simulink library "pmm"  (R2021b)
settings: Solver=VariableStepAuto  StartTime=0.0  StopTime=10.0  RelTol=1e-3
undefined symbols (not defined in the file): APMM_CoolgFanActCurr_X_pct, APMM_EWP1Curr_X_c, APMM_EWP3Curr_X_c, APMM_LVBattChktime_X_enum, APMM_LVBattChrgtime_X_enum, APMM_LVChrgLv_X_mV, ENUM_ANTITHEFT_ALARM, ENUM_ANTITHEFT_ARM, ENUM_ANTITHEFT_DISARM, ENUM_ANTITHEFT_WAIT, ENUM_APSSYSTEMSTA_REMOTEACTIVE, ENUM_CHRGPLUGSTA_NONE, ENUM_CRASHSTATE_FRONTFIRSTLV, ENUM_CRASHSTATE_LEFTSIDE, ENUM_CRASHSTATE_RIGHTSIDE, ENUM_DRIVETRAIN_AWD, ENUM_DRIVETRAIN_FWD, ENUM_DRIVETRAIN_RWD, ENUM_DRSEATSTA_EMPTY, ENUM_DRSEATSTA_INVALID, ENUM_DRSEATSTA_OCCUPIED, ENUM_EPBSTA_APPLIED, ENUM_GEARACTUALPOSN_D, ENUM_GEARACTUALPOSN_N, ENUM_GEARACTUALPOSN_P, ENUM_GEARACTUALPOSN_R, ENUM_HVBATTREADYPRE_READY, ENUM_OTACHKSTA_NOREQUEST, ENUM_OTACHKSTA_NOTIMEOUT, ENUM_OTACHKSTA_TIMEOUT, ENUM_PDKEYRAWLULOCK_INLOCK, ENUM_PDKEYRAWLULOCK_INUNLOCK, ENUM_PDKEYRAWPS_INPS, ENUM_PDKEYSTA_LOCK, ENUM_PDKEYSTA_PS, ENUM_PDKEYSTA_UNAVALIABLE, ENUM_PDKEYSTA_UNLOCK, ENUM_POWERSTA_OFF, ENUM_POWERSTA_OFFC, ENUM_POWERSTA_STANDBY, ENUM_PWRREQOTA_NOREQUEST, ENUM_PWRREQOTA_REQPOWEROFF, ENUM_PWRREQOTA_REQPOWERSTDBY, ENUM_PWRSTASW_READY, ENUM_V2LSTA_NOPLUG, ENUM_VEHICLETYPE_D31L24, ENUM_VEHMALFUNLEVEL_LEVEL3, ENUM_VEHMALFUNLEVEL_LEVEL4, FALSE, KPMM_AllDoorClosedHoldTime_s, KPMM_APSAllowThd_pct, KPMM_BattDownFailtime_s, KPMM_BattUpFailtime_s, KPMM_BattUpResetRty_cnt, KPMM_BattUpResetSW_flg, KPMM_BattUpResetTO_s, KPMM_BattUpRstDlyTO_s, KPMM_BrakeSWHoldTime_s, KPMM_CANValidChkFailtime_s, KPMM_ChrgPlugHoldTime_s ... (+87)
libraries: simulink x29, hcu_lib x24
(part 4 of 7)

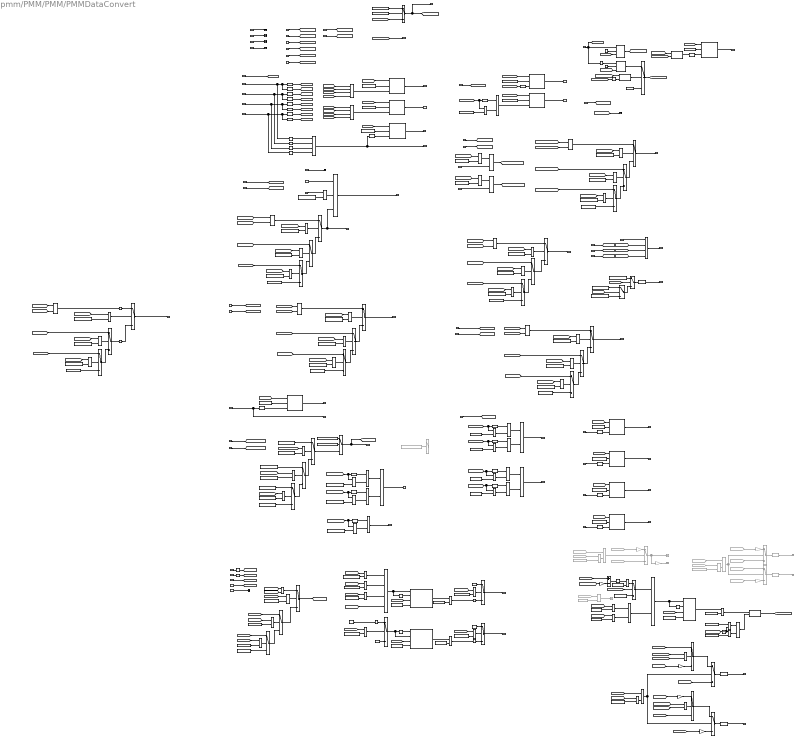
== system pmm/PMM/PMM/PMMDataConvert ==
  note: Detect HV power state
  note: Detect PW Continue Use
  note: Detect SchedChgwake
  note: Detect IVI Power OFF
  note: Monitor for DCDC fault level
  note: Safety Check
  note: 0 = HVIL close; 1 = HVIL open
  note: Seat Switch Rising Edge
  note: Detect Gun Plug Rising/Faling Edge
  note: KEY STATE
  note: Brake signal convert to rising edge
  note: Door judgement
  note: Precharge Check
  note: MCU Enable
  note: MCU Discharge
  note: MCU Ready
  note: Antitheft State
  note: OPDS Signal tramsmit function
  note: BMSWarn judgement
  note: MCU DC Bus Max Voltage judgement
  note: VPMM_SafetyChkHLv_flg
      | 0 Fail
      | 1 OK
  note: VPMM_TMSpdThdSta_flg
      | 0 = Not allow MCU disable
      | 1 = Allow MCU disable
  note: 0 = No fail;
      | 1 = fail
  note: VPMM_SafetyChkMLv_flg
      | 0 Fail
      | 1 OK
  note: Aux Battery Handle
  note: Comment out to reduce CPU resource.
      | Use below if judgement to avoid float multiply.
  note: MCU Disable
  task_time_s : Inport
  VBCM_AntitheftSta_enum : Inport  Port=2
  VINP_DrDoorSW_flg : Inport  Port=3
  VINP_PsDoorSW_flg : Inport  Port=4
  VINP_RRDoorSW_flg : Inport  Port=5
  VINP_RLDoorSW_flg : Inport  Port=6
  VINP_BrakeSWGPIO_flg : Inport  Port=7
  VINP_FrMCUDCBusVolt_V : Inport  Port=8
  VINP_FrMCUDischrgSta_flg : Inport  Port=9
  VINP_FrMCUEnaSta_flg : Inport  Port=10
  VINP_FrMCUErr_enum : Inport  Port=11
  VINP_FrMCUReady4Pre_flg : Inport  Port=12
  VINP_FrMCUReady_flg : Inport  Port=13
  VINP_FrMCUTemp_C : Inport  Port=14
  VINP_RrMCUDCBusVolt_V : Inport  Port=15
  VINP_RrMCUDischrgSta_flg : Inport  Port=16
  VINP_RrMCUEnaSta_flg : Inport  Port=17
  VINP_RrMCUErr_enum : Inport  Port=18
  VINP_RrMCUReady4Pre_flg : Inport  Port=19
  VINP_RrMCUReady_flg : Inport  Port=20
  VINP_RrMCUTemp_C : Inport  Port=21
  VINP_DCDCReady4Pre_flg : Inport  Port=22
  VINP_OBCReady4Pre_flg : Inport  Port=23
  VINP_HVBattReady4Pre_enum : Inport  Port=24
  VINP_PDKeyAreaPS_enum : Inport  Port=25
  VINP_PDKeyAreaLockUnlock_enum : Inport  Port=26
  VINP_ChrgPlugSta_enum : Inport  Port=27
  VINP_SeatSW_flg : Inport  Port=28
  VINP_HVILSta_flg : Inport  Port=29
  VINP_CrashOutputSts_enum : Inport  Port=30
  VPMM_PowerSta_enum : Inport  Port=31
  VINP_RrTMSpd_rpm : Inport  Port=32
  VINP_FrTMSpd_rpm : Inport  Port=33
  VINP_BMSWarn5_flg : Inport  Port=34
  VINP_BMSWarn6_flg : Inport  Port=35
  VINP_BMSWarn7_flg : Inport  Port=36
  VINP_BMSWarn8_flg : Inport  Port=37
  VINP_DrivetrainSelect_enum : Inport  Port=38
  VINP_DCDCFaultSta_enum : Inport  Port=39
  VINP_IVIPwroffreq_flg : Inport  Port=40
  VINP_SchedChgwake_flg : Inport  Port=41
  VINP_PWCONTINUEUSE_flg : Inport  Port=42
  VPMM_HVPwrSta_flg : Inport  Port=43
  VINP_LVBattDet12V_V : Inport  Port=44
  VINP_AuxBattVolmV_mV : Inport  Port=45
  VINP_NewNMSpec_flg : Inport  Port=46
  VINP_VehicleType_enum : Inport  Port=47
  VINP_CANMsgValidBMS5_flg : Inport  Port=48
  VTQD_CrashDetd_flg : Inport  Port=49
  VDDM_DrStSWCFS_flg : Inport  Port=50
  AND{,3..6,8} (6 alike) : Logic  AllPortsSameDT=off  OutDataTypeStr=boolean
  AND1 : Logic  Inputs=3  AllPortsSameDT=off  OutDataTypeStr=boolean
  AND2 : Logic  Operator=OR  AllPortsSameDT=off  OutDataTypeStr=boolean
  AND7 : Logic  Operator=OR  Inputs=4  AllPortsSameDT=off  OutDataTypeStr=boolean
  Abs : Abs
  Abs1 : Abs
  Abs2 : Abs
  Add : Sum  Inputs=+-
  Constant : Constant  Value=KPMM_DoorSWHoldTime_s
  Constant1 : Constant  Value=KPMM_DoorSWHoldTime_s
  Constant10 : Constant  Commented=on  Value=ENUM_VEHICLETYPE_D31L24
  Constant{4,11,19,22,30,38,84} (7 alike) : Constant  Value=ENUM_DRIVETRAIN_AWD
  Constant12 : Constant  Commented=on  Value=ENUM_VEHICLETYPE_D31L24
  Constant{6,13,21,32,39,46,85} (7 alike) : Constant  Value=ENUM_DRIVETRAIN_FWD
  Constant14 : Constant  Value=ENUM_HVBATTREADYPRE_READY
  Constant{8,15,23,34,40,51,86} (7 alike) : Constant  Value=ENUM_DRIVETRAIN_RWD
  Constant{7,9,16..17,28,55,82,87,93} (9 alike) : Constant  Value=FALSE
  Constant18 : Constant  Value=KPMM_ChrgPlugHoldTime_s
  Constant2 : Constant  Value=ZERO_FLOAT
  Constant20 : Constant  Value=KPMM_ChrgPlugHoldTime_s
  Constant24 : Constant  Value=KPMM_RrMCUDischrgVolt_V
  Constant25 : Constant  Value=KPMM_FrMCUDischrgVolt_V
  Constant26 : Constant  Value=KPMM_DrivetrainSelect_enum_ovrdflg
  Constant27 : Constant  Commented=on  Value=FALSE
  Constant29 : Constant  Value=ENUM_VEHICLETYPE_D31L24
  Constant3 : Constant  Value=KPMM_SeatSWHoldTime_s
  Constant31 : Constant  Value=ENUM_CHRGPLUGSTA_NONE
  Constant33 : Constant  Value=KPMM_LVADCUpThd_mV  OutDataTypeStr=uint16
  Constant35 : Constant  Value=ENUM_POWERSTA_STANDBY  OutDataTypeStr=uint8
  Constant36 : Constant  Value=KPMM_LVADCDiffThd_mV  OutDataTypeStr=uint16
  Constant37 : Constant  Value=KPMM_AllDoorClosedHoldTime_s
  Constant41 : Constant  Value=KPMM_BrakeSWHoldTime_s
  Constant42 : Constant  Value=KPMM_PDKeySta_enum_ovrdval
  Constant43 : Constant  Value=ENUM_PDKEYRAWPS_INPS
  Constant44 : Constant  Value=KPMM_PDKeySta_enum_ovrdflg
  Constant45 : Constant  Value=ENUM_PDKEYRAWLULOCK_INUNLOCK
  Constant47 : Constant  Value=ENUM_PDKEYRAWLULOCK_INLOCK
  Constant48 : Constant  Value=ENUM_PDKEYSTA_UNAVALIABLE
  Constant49 : Constant  Value=ENUM_PDKEYSTA_LOCK
  Constant5 : Constant  Value=ENUM_CRASHSTATE_FRONTFIRSTLV
  Constant50 : Constant  Value=ENUM_PDKEYSTA_UNLOCK
  Constant52 : Constant  Value=KPMM_DrivetrainSelect_enum_ovrdval
  Constant53 : Constant  Value=ENUM_ANTITHEFT_DISARM
  Constant54 : Constant  Value=ENUM_ANTITHEFT_WAIT
  Constant56 : Constant  Value=ENUM_PDKEYSTA_PS
  Constant57 : Constant  Value=KPMM_LVADCLoThd_mV  OutDataTypeStr=uint16
  Constant58 : Constant  Value=ENUM_PDKEYSTA_UNLOCK
  Constant59 : Constant  Value=ENUM_PDKEYSTA_PS
  Constant60 : Constant  Value=ENUM_ANTITHEFT_ARM
  Constant61 : Constant  Value=ENUM_ANTITHEFT_ALARM
  Constant62 : Constant  Value=ENUM_PDKEYSTA_LOCK
  Constant63 : Constant  Value=KPMM_IVIPwroffHoldTime_s
  Constant64 : Constant  Value=KPMM_SchedChgHoldTime_s
  Constant65 : Constant  Value=KPMM_PWCONTINUEHoldTime_s
  Constant66 : Constant  Value=KPMM_HVPwrStaHoldTime_s
  Constant67 : Constant  Value=ENUM_CRASHSTATE_RIGHTSIDE
  Constant68 : Constant  Value=ENUM_CRASHSTATE_LEFTSIDE
  Constant69 : Constant  Value=KPMM_TMSpdMCUDisThrsh_rpm
  Constant70 : Constant  Value=TRUE
  Constant71 : Constant  Value=KPMM_SaftyChkHLvTO_s
  Constant72 : Constant  Value=ENUM_POWERSTA_OFF
  Constant73 : Constant  Value=TRUE
  Constant74 : Constant  Value=KPMM_SaftyChkMLvTO_s
  Constant75 : Constant  Value=KPMM_SaftyChkMLvTO_s
  Constant76 : Constant  Value=TRUE
  Constant77 : Constant  Value=ENUM_POWERSTA_OFF
  Constant78 : Constant  Value=KPMM_LVADCErrTO_s  OutDataTypeStr=single
  Constant79 : Constant  Value=KPMM_SaftyChkHLvTO_s
  Constant80 : Constant  Value=ENUM_POWERSTA_OFF  OutDataTypeStr=uint8
  Constant81 : Constant  Commented=on  Value=0xFFFF  OutDataTypeStr=uint16
  Constant83 : Constant  Value=KPMM_LVADCErrTO_s  OutDataTypeStr=single
  Constant88 : Constant  Value=ENUM_DRSEATSTA_OCCUPIED
  Constant89 : Constant  Value=ENUM_DRSEATSTA_EMPTY
  Constant90 : Constant  Value=ENUM_DRSEATSTA_INVALID
  Constant91 : Constant  Value=200
  Constant92 : Constant  Value=2000
  Data Type Conversion : DataTypeConversion  OutDataTypeStr=uint8
  Data Type Conversion1 : DataTypeConversion  Commented=on
  Data Type Conversion2 : DataTypeConversion
  Data Type Conversion3 : DataTypeConversion  Commented=on
  Data Type Conversion4 : DataTypeConversion
  Delay : Delay  DelayLength=1
  DelayEnable : hcu_lib/Basic_Blocks/DelayEnable
  DelayEnable1 : hcu_lib/Basic_Blocks/DelayEnable
  Detect Change{,1..6} (7 alike) : simulink/Logic and Bit Operations/Detect Change  vinit=0  OutDataTypeStr=boolean
  Detect Decrease{,1..4} (5 alike) : simulink/Logic and Bit Operations/Detect Decrease  vinit=0.0  OutDataTypeStr=boolean
  Detect Increase{,1..11} (12 alike) : simulink/Logic and Bit Operations/Detect Increase  vinit=0.0  OutDataTypeStr=boolean
  Equal{,1..9,12,14..18,20..22,24..25,27..38,41,44,50..52} (38 alike) : RelationalOperator  Operator===  OutDataTypeStr=boolean  RndMeth=Simplest
  Equal10 : RelationalOperator  Operator=<=  OutDataTypeStr=boolean  RndMeth=Simplest
  Equal11 : RelationalOperator  Operator=<=  OutDataTypeStr=boolean  RndMeth=Simplest
  Equal13 : RelationalOperator  Commented=on  Operator=~=  OutDataTypeStr=boolean  RndMeth=Simplest
  Equal19 : RelationalOperator  Operator=~=  OutDataTypeStr=boolean  RndMeth=Simplest
  Equal23 : RelationalOperator  Commented=on  Operator===  OutDataTypeStr=boolean  RndMeth=Simplest
  Equal26 : RelationalOperator  Commented=on  Operator=~=  OutDataTypeStr=boolean  RndMeth=Simplest
  Equal{39..40,42,47..48} (5 alike) : RelationalOperator  OutDataTypeStr=boolean  RndMeth=Simplest
  Equal43 : RelationalOperator  Operator=<  OutDataTypeStr=boolean  RndMeth=Simplest
  Equal45 : RelationalOperator  Operator=~=  OutDataTypeStr=boolean  RndMeth=Simplest
  Equal46 : RelationalOperator  Operator=~=  OutDataTypeStr=boolean  RndMeth=Simplest
  Equal49 : RelationalOperator  Operator=<=  OutDataTypeStr=boolean  RndMeth=Simplest
  From100 : From  Commented=on  GotoTag=VINP_LVBattDet12V_V
  From{95,101..102,117} (4 alike) : From  Commented=on  GotoTag=VINP_AuxBattVolmV_mV
  From93 : From  Commented=on  GotoTag=VINP_VehicleType_enum
  From94 : From  Commented=on  GotoTag=VINP_NewNMSpec_flg
  From96 : From  Commented=on  GotoTag=VINP_LVBattDet12V_V
  From97 : From  Commented=on  GotoTag=VINP_VehicleType_enum
  From98 : From  Commented=on  GotoTag=VINP_NewNMSpec_flg
  From99 : From  Commented=on  GotoTag=VINP_LVBattDet12V_V
  Gain : Gain  Commented=on  Gain=1000
  Gain1 : Gain  Commented=on  Gain=0.001
  Gain2 : Gain  Commented=on  Gain=0.001
  Gain3 : Gain  Commented=on  Gain=1000
  Gain4 : Gain  Gain=1000
  Gain5 : Gain  Gain=0.001
  Gain6 : Gain  Gain=1000
  Gain7 : Gain  Gain=1000
  Hold{,1..10} (11 alike) : hcu_lib/Basic_Blocks/Hold  SystemSampleTime=-1  VariantActivationTime=update diagram  Latency=0  AutoFrameSizeCalculation=off
      settings: SourceProductName=HCU Relative Block Library
  LiuzgSwitch{1..18,22..32} (29 alike) : Switch  Criteria=u2 ~= 0
      settings: AttributesFormatString=<%<Criteria>>
  LiuzgSwitch19 : Switch  Commented=on  Criteria=u2 ~= 0
      settings: AttributesFormatString=<%<Criteria>>
  LiuzgSwitch20 : Switch  Commented=on  Criteria=u2 ~= 0
      settings: AttributesFormatString=<%<Criteria>>
  LiuzgSwitch21 : Switch  Commented=on  Criteria=u2 ~= 0
      settings: AttributesFormatString=<%<Criteria>>
  Logical Operator : Logic  Operator=NOT  AllPortsSameDT=off  OutDataTypeStr=boolean
  Logical Operator{1..3,5..6,8..9,11,15..17,20} (12 alike) : Logic  AllPortsSameDT=off  OutDataTypeStr=boolean
  Logical Operator{4,7,10,18..19} (5 alike) : Logic  Operator=OR  AllPortsSameDT=off  OutDataTypeStr=boolean
  Logical Operator12 : Logic  Commented=on  AllPortsSameDT=off  OutDataTypeStr=boolean
  Logical Operator13 : Logic  Operator=OR  Inputs=4  AllPortsSameDT=off  OutDataTypeStr=boolean
  Logical Operator14 : Logic  Commented=on  AllPortsSameDT=off  OutDataTypeStr=boolean
  Logical Operator21 : Logic  Operator=NOT  AllPortsSameDT=off  OutDataTypeStr=boolean
  Logical Operator22 : Logic  Operator=NOT  AllPortsSameDT=off  OutDataTypeStr=boolean
  Max : MinMax  Function=max  Inputs=2
  Max1 : MinMax  Function=max  Inputs=2
  NOT{1..9,11} (10 alike) : Logic  Operator=NOT  AllPortsSameDT=off  OutDataTypeStr=boolean
  OR : Logic  Operator=OR  Inputs=4  AllPortsSameDT=off  OutDataTypeStr=boolean
  OR1 : Logic  Operator=OR  Inputs=4  AllPortsSameDT=off  OutDataTypeStr=boolean
  OR2 : Logic  Inputs=4  AllPortsSameDT=off  OutDataTypeStr=boolean
  SR_Latch : hcu_lib/Basic_Blocks/SR_Latch
  SR_Latch1 : hcu_lib/Basic_Blocks/SR_Latch
  SR_Latch2 : hcu_lib/Basic_Blocks/SR_Latch
  Switch{,2..4} (4 alike) : Switch  Criteria=u2 ~= 0
      Switch2 settings: AttributesFormatString=%<Criteria>
      Switch3 settings: AttributesFormatString=%<Criteria>
  Switch1 : Switch  Commented=on  Criteria=u2 ~= 0
  Switch5 : Switch  Criteria=u2 > Threshold
  Switch7 : Switch  Criteria=u2 ~= 0  Threshold=15
  Switch8 : Switch  Criteria=u2 ~= 0  Threshold=15
  Switch9 : Switch  Criteria=u2 ~= 0  Threshold=10.9
  Terminator{,1..6} (7 alike) : Terminator
  Terminator7 : Terminator  Commented=on
  Terminator8 : Terminator  Commented=on
  Terminator9 : Terminator  Commented=on
  Timer : hcu_lib/Basic_Blocks/Timer
  Timer1 : hcu_lib/Basic_Blocks/Timer
  Timer2 : hcu_lib/Basic_Blocks/Test Detection Criteria/Timer
  Unit Delay2 : UnitDelay  SampleTime=-1  HasFrameUpgradeWarning=on
  VPMM_AuxBatVolt_V_commentout : Terminator  Commented=on
  VPMM_AuxBatVolt_mV_commentout : Terminator  Commented=on
  VPMM_DetectDoorOpened_flg : Outport
  VPMM_DetectDoorClosed_flg : Outport  Port=2
  VPMM_BrkPedalPressed_flg : Outport  Port=3
  VPMM_PreChrgChk_flg : Outport  Port=4
  VPMM_AllDoorClosed_flg : Outport  Port=5
  VPMM_MCUEnable_flg : Outport  Port=6
  VPMM_MCUDischrgFinished_flg : Outport  Port=7
  VPMM_MCUReady_flg : Outport  Port=8
  VPMM_PDKeySta_enum : Outport  Port=9
  VPMM_BrkPedalRisingEdge_flg : Outport  Port=10
  VPMM_AllDoorCloseRisingEdge_flg : Outport  Port=11
  VPMM_DrivetrainSelect_enum : Outport  Port=12
  VPMM_ChrgPlugInRisingEdge_flg : Outport  Port=13
  VPMM_ChrgPlugOutFallingEdge_flg : Outport  Port=14
  VPMM_SeatSWRisingEdge_flg : Outport  Port=15
  VPMM_SafetyChkMLv_flg : Outport  Port=16
  VPMM_SafetyChkHLv_flg : Outport  Port=17
  VPMM_DrSeatSta_enum : Outport  Port=18
  VPMM_BMSWarm_flg : Outport  Port=19
  VPMM_MCUDCBusMaxVolt_V : Outport  Port=20
  VPMM_DetectAntitheftUnlock_flg : Outport  Port=21
  VPMM_DetectPDKeyUnlock_flg : Outport  Port=22
  VPMM_DetectAntitheftLock_flg : Outport  Port=23
  VPMM_DetectPDKeyLock_flg : Outport  Port=24
  VPMM_DetectIVIPwroffreq_flg : Outport  Port=25
  VPMM_DetectSchedChg_flg : Outport  Port=26
  VPMM_DetectPWCONTINUE_flg : Outport  Port=27
  VPMM_DetectHVPwrSta_flg : Outport  Port=28
  VPMM_MCUReady4Pre_flg : Outport  Port=29
  VPMM_AuxBatVolt_mV : Outport  Port=30
  VPMM_AuxBatVolt_V : Outport  Port=31
  VPMM_ADCStaChkFail_flg : Outport  Port=32
  VPMM_MCUDisable_flg : Outport  Port=33
  wires:
  Data Type Conversion/1 -> VPMM_DrSeatSta_enum/1  "VPMM_DrSeatSta_enum"
  [VPMM_FrMCUDCBusVolt_V] -> Max1/2
  [VPMM_RrMCUDCBusVolt_V] -> Max1/1
  [VPMM_FrMCUDCBusVolt_V] -> LiuzgSwitch18/1
  Max1/1 -> LiuzgSwitch25/1
  Constant7/1 -> LiuzgSwitch26/3
  Constant46/1 -> Equal30/2
  LiuzgSwitch26/1 -> LiuzgSwitch18/3
  Equal12/1 -> LiuzgSwitch25/2
  Constant51/1 -> Equal31/2
  [VPMM_DrivetrainSelect_enum] -> Equal12/1
  Equal30/1 -> LiuzgSwitch18/2
  Constant22/1 -> Equal12/2
  LiuzgSwitch18/1 -> LiuzgSwitch25/3
  [VPMM_DrivetrainSelect_enum] -> Equal30/1
  Equal31/1 -> LiuzgSwitch26/2
  [VPMM_DrivetrainSelect_enum] -> Equal31/1
  [VPMM_RrMCUDCBusVolt_V] -> LiuzgSwitch26/1
  LiuzgSwitch25/1 -> VPMM_MCUDCBusMaxVolt_V/1  "VPMM_MCUDCBusMaxVolt_V"
  [VPMM_FrMCUDCBusVolt_V] -> Equal11/1
  [VPMM_RrMCUDCBusVolt_V] -> Equal10/1
  VINP_BMSWarn5_flg/1 -> AND7/1
  AND7/1 -> VPMM_BMSWarm_flg/1  "VPMM_BMSWarm_flg"
  Abs1/1 -> [VINP_FrTMSpdABS_rpm]
  Abs/1 -> [VINP_RrTMSpdABS_rpm]
  LiuzgSwitch23/1 -> [VPMM_TMSpd_rpm]  "VPMM_TMSpd_rpm"
  Constant2/1 -> LiuzgSwitch24/3
  Max/1 -> LiuzgSwitch23/1
  [VINP_FrTMSpdABS_rpm] -> Max/2
  [VINP_RrTMSpdABS_rpm] -> Max/1
  LiuzgSwitch22/1 -> LiuzgSwitch23/3
  LiuzgSwitch24/1 -> LiuzgSwitch22/3
  [VINP_FrTMSpdABS_rpm] -> LiuzgSwitch22/1
  [VINP_RrTMSpdABS_rpm] -> LiuzgSwitch24/1
  [VPMM_DrivetrainSelect_enum] -> Equal27/1
  Constant40/1 -> Equal29/2
  Constant38/1 -> Equal27/2
  Equal29/1 -> LiuzgSwitch24/2
  Equal27/1 -> LiuzgSwitch23/2
  Constant39/1 -> Equal28/2
  [VPMM_DrivetrainSelect_enum] -> Equal29/1
  Equal28/1 -> LiuzgSwitch22/2
  [VPMM_DrivetrainSelect_enum] -> Equal28/1
  VINP_FrTMSpd_rpm/1 -> Abs1/1
  VINP_RrTMSpd_rpm/1 -> Abs/1
  VPMM_PowerSta_enum/1 -> [VPMM_PowerSta_enum]
  [task_time_s] -> Hold4/1
  Hold4/1 -> VPMM_SeatSWRisingEdge_flg/1  "VPMM_SeatSWRisingEdge_flg"
  VINP_SeatSW_flg/1 -> [VPMM_SeatSW_flg], Logical Operator/1, DelayEnable/1
  Constant3/1 -> Hold4/2
  Detect Increase6/1 -> Hold4/3
  Constant18/1 -> Hold6/2
  Hold5/1 -> VPMM_ChrgPlugOutFallingEdge_flg/1  "VPMM_ChrgPlugOutFallingEdge_flg"
  Detect Increase7/1 -> Hold6/3
  [VINP_ChrgPlugSta_enum] -> Detect Increase7/1
  [task_time_s] -> Hold5/1
  VINP_ChrgPlugSta_enum/1 -> [VINP_ChrgPlugSta_enum]
  Constant20/1 -> Hold5/2
  [task_time_s] -> Hold6/1
  Logical Operator1/1 -> Hold5/3
  Hold6/1 -> VPMM_ChrgPlugInRisingEdge_flg/1  "VPMM_ChrgPlugInRisingEdge_flg"
  Equal25/1 -> Logical Operator1/2
  [VINP_ChrgPlugSta_enum] -> Detect Decrease4/1, Equal25/1
  Constant31/1 -> Equal25/2
  Detect Decrease4/1 -> Logical Operator1/1
  Equal24/1 -> AND1/2
  Constant14/1 -> Equal24/2
  Switch/1 -> VPMM_DrivetrainSelect_enum/1, [VPMM_DrivetrainSelect_enum]  "VPMM_DrivetrainSelect_enum"
  Detect Increase5/1 -> Hold2/3
  Hold2/1 -> VPMM_AllDoorCloseRisingEdge_flg/1  "VPMM_AllDoorCloseRisingEdge_flg"
  Constant37/1 -> Hold2/2
  [task_time_s] -> Hold2/1
  VINP_OBCReady4Pre_flg/1 -> Terminator1/1
  VINP_HVBattReady4Pre_enum/1 -> Equal24/1
  Constant50/1 -> LiuzgSwitch13/1
  Constant56/1 -> LiuzgSwitch14/1
  Constant49/1 -> LiuzgSwitch15/1
  [VINP_PDKeyAreaLockUnlock_enum] -> Equal22/1
  Equal22/1 -> LiuzgSwitch15/2
  [VINP_PDKeyAreaLockUnlock_enum] -> Equal21/1
  LiuzgSwitch13/1 -> LiuzgSwitch14/3
  Constant43/1 -> Equal20/2
  Equal21/1 -> LiuzgSwitch13/2
  [VINP_PDKeyAreaPS_enum] -> Equal20/1
  Constant47/1 -> Equal22/2
  Equal20/1 -> LiuzgSwitch14/2
  LiuzgSwitch15/1 -> LiuzgSwitch13/3
  Constant45/1 -> Equal21/2
  Constant48/1 -> LiuzgSwitch15/3
  VINP_PDKeyAreaPS_enum/1 -> [VINP_PDKeyAreaPS_enum]
  Hold3/1 -> VPMM_BrkPedalRisingEdge_flg/1  "VPMM_BrkPedalRisingEdge_flg"
  [task_time_s] -> Hold3/1
  Constant41/1 -> Hold3/2
  Detect Increase4/1 -> Hold3/3  "VPMM_BrakePaddleRisingEdge_flg"
  [VPMM_DrivetrainSelect_enum] -> Equal15/1
  LiuzgSwitch10/1 -> LiuzgSwitch11/3
  LiuzgSwitch11/1 -> VPMM_MCUReady_flg/1  "VPMM_MCUReady_flg"
  [VINP_RrMCUReady_flg] -> LiuzgSwitch12/1
  Constant30/1 -> Equal14/2
  Constant28/1 -> LiuzgSwitch12/3
  Equal16/1 -> LiuzgSwitch12/2
  [VPMM_DrivetrainSelect_enum] -> Equal16/1
  AND8/1 -> LiuzgSwitch11/1
  [VINP_FrMCUReady_flg] -> AND8/1
  [VPMM_DrivetrainSelect_enum] -> Equal14/1
  Constant34/1 -> Equal16/2
  LiuzgSwitch12/1 -> LiuzgSwitch10/3
  VINP_RrMCUReady_flg/1 -> [VINP_RrMCUReady_flg]
  Constant32/1 -> Equal15/2
  [VINP_FrMCUReady_flg] -> LiuzgSwitch10/1
  VINP_FrMCUReady_flg/1 -> [VINP_FrMCUReady_flg]
  [VINP_RrMCUReady_flg] -> AND8/2
  Equal14/1 -> LiuzgSwitch11/2
  Equal15/1 -> LiuzgSwitch10/2
  VINP_RrMCUTemp_C/1 -> Terminator5/1
  VINP_RrMCUErr_enum/1 -> Terminator3/1
  VINP_FrMCUTemp_C/1 -> Terminator2/1
  VINP_FrMCUErr_enum/1 -> Terminator/1
  LiuzgSwitch8/1 -> VPMM_MCUDischrgFinished_flg/1  "VPMM_MCUDischrgFinished_flg"
  [VINP_RrDischrgComplete_flg] -> AND4/2
  [VINP_FrDischrgComplete_flg] -> AND4/1
  AND6/1 -> [VINP_FrDischrgComplete_flg]
  AND5/1 -> [VINP_RrDischrgComplete_flg]
  VINP_FrMCUDCBusVolt_V/1 -> [VPMM_FrMCUDCBusVolt_V]
  Constant25/1 -> Equal11/2
  Equal11/1 -> AND6/1
  VINP_FrMCUDischrgSta_flg/1 -> AND6/2
  VINP_RrMCUDischrgSta_flg/1 -> AND5/2
  Equal10/1 -> AND5/1
  Constant24/1 -> Equal10/2
  VINP_RrMCUDCBusVolt_V/1 -> [VPMM_RrMCUDCBusVolt_V]
  [VINP_RrDischrgComplete_flg] -> LiuzgSwitch9/1
  [VPMM_DrivetrainSelect_enum] -> Equal9/1
  Equal9/1 -> LiuzgSwitch9/2
  [VPMM_DrivetrainSelect_enum] -> Equal8/1
  LiuzgSwitch7/1 -> LiuzgSwitch8/3
  Constant19/1 -> Equal4/2
  Equal8/1 -> LiuzgSwitch7/2
  [VPMM_DrivetrainSelect_enum] -> Equal4/1
  Constant23/1 -> Equal9/2
  Equal4/1 -> LiuzgSwitch8/2
  LiuzgSwitch9/1 -> LiuzgSwitch7/3
  Constant21/1 -> Equal8/2
  Constant17/1 -> LiuzgSwitch9/3
  AND4/1 -> LiuzgSwitch8/1
  [VINP_FrDischrgComplete_flg] -> LiuzgSwitch7/1
  [VINP_RrMCUEnaSta_flg] -> AND3/2
  [VINP_FrMCUEnaSta_flg] -> AND3/1
  VINP_RrMCUEnaSta_flg/1 -> [VINP_RrMCUEnaSta_flg]
  VINP_FrMCUEnaSta_flg/1 -> [VINP_FrMCUEnaSta_flg]
  [VINP_FrMCUEnaSta_flg] -> LiuzgSwitch1/1
  AND3/1 -> LiuzgSwitch2/1
  Constant16/1 -> LiuzgSwitch3/3
  Constant6/1 -> Equal2/2
  LiuzgSwitch3/1 -> LiuzgSwitch1/3
  Equal1/1 -> LiuzgSwitch2/2
  Constant8/1 -> Equal3/2
  [VPMM_DrivetrainSelect_enum] -> Equal1/1
  Equal2/1 -> LiuzgSwitch1/2
  Constant4/1 -> Equal1/2
  LiuzgSwitch2/1 -> VPMM_MCUEnable_flg/1  "VPMM_MCUEnable_flg"
  LiuzgSwitch1/1 -> LiuzgSwitch2/3
  [VPMM_DrivetrainSelect_enum] -> Equal2/1
  Equal3/1 -> LiuzgSwitch3/2
  [VPMM_DrivetrainSelect_enum] -> Equal3/1
  [VINP_RrMCUEnaSta_flg] -> LiuzgSwitch3/1
  OR2/1 -> VPMM_AllDoorClosed_flg/1, Detect Increase5/1  "VPMM_AllDoorClosed_flg"
  NOT5/1 -> OR2/4
  NOT4/1 -> OR2/3
  NOT3/1 -> OR2/2
  NOT2/1 -> OR2/1
  AND1/1 -> VPMM_PreChrgChk_flg/1  "VPMM_PreChrgChk_flg"
  VINP_DCDCReady4Pre_flg/1 -> AND1/1
  LiuzgSwitch5/1 -> VPMM_MCUReady4Pre_flg/1, AND1/3  "VPMM_MCUReady4Pre_flg"
  [VINP_FrMCUReady4Pre_flg] -> AND/2
  [VINP_RrMCUReady4Pre_flg] -> AND/1
  VINP_FrMCUReady4Pre_flg/1 -> [VINP_FrMCUReady4Pre_flg]
  VINP_RrMCUReady4Pre_flg/1 -> [VINP_RrMCUReady4Pre_flg]
  [VINP_RrMCUReady4Pre_flg] -> LiuzgSwitch6/1
  [VPMM_DrivetrainSelect_enum] -> Equal6/1
  Equal6/1 -> LiuzgSwitch4/2
  [VINP_FrMCUReady4Pre_flg] -> LiuzgSwitch4/1
  Equal7/1 -> LiuzgSwitch6/2
  LiuzgSwitch4/1 -> LiuzgSwitch5/3
  [VPMM_DrivetrainSelect_enum] -> Equal7/1
  Constant11/1 -> Equal5/2
  Constant15/1 -> Equal7/2
  LiuzgSwitch6/1 -> LiuzgSwitch4/3
  AND/1 -> LiuzgSwitch5/1
  Constant13/1 -> Equal6/2
  Equal5/1 -> LiuzgSwitch5/2
  [VPMM_DrivetrainSelect_enum] -> Equal5/1
  Constant9/1 -> LiuzgSwitch6/3
  VINP_BrakeSWGPIO_flg/1 -> Detect Increase4/1, VPMM_BrkPedalPressed_flg/1
  [VPMM_FlClosed_flg] -> OR1/1
  [VPMM_FrClosed_flg] -> OR1/2
  [VPMM_RlClosed_flg] -> OR1/3
  [VPMM_RrClosed_flg] -> OR1/4
  Hold1/1 -> VPMM_DetectDoorClosed_flg/1  "VPMM_DetectDoorClosed_flg"
  OR1/1 -> Hold1/3
  [task_time_s] -> Hold1/1
  Constant1/1 -> Hold1/2
  Hold/1 -> VPMM_DetectDoorOpened_flg/1  "VPMM_DetectDoorOpened_flg"
  Constant/1 -> Hold/2
  [task_time_s] -> Hold/1
  OR/1 -> Hold/3
  task_time_s/1 -> [task_time_s]
  [VPMM_RrOpened_flg] -> OR/4
  [VPMM_RlOpened_flg] -> OR/3
  [VPMM_FlOpened_flg] -> OR/1
  [VPMM_FrOpened_flg] -> OR/2
  Detect Decrease3/1 -> [VPMM_RrClosed_flg]
  Detect Increase3/1 -> [VPMM_RrOpened_flg]
  Detect Decrease2/1 -> [VPMM_RlClosed_flg]
  Detect Increase2/1 -> [VPMM_RlOpened_flg]
  Detect Decrease1/1 -> [VPMM_FrClosed_flg]
  Detect Increase1/1 -> [VPMM_FrOpened_flg]
  Detect Decrease/1 -> [VPMM_FlClosed_flg]
  Detect Increase/1 -> [VPMM_FlOpened_flg]
  VINP_RLDoorSW_flg/1 -> Detect Increase3/1, Detect Decrease3/1, NOT5/1
  VINP_RRDoorSW_flg/1 -> Detect Increase2/1, Detect Decrease2/1, NOT4/1
  VINP_PsDoorSW_flg/1 -> Detect Increase1/1, Detect Decrease1/1, NOT3/1
  VINP_DrDoorSW_flg/1 -> Detect Increase/1, Detect Decrease/1, NOT2/1
  Constant26/1 -> Switch/2
  VINP_DrivetrainSelect_enum/1 -> [VINP_DrivetrainSelect_enum]
  [VINP_DrivetrainSelect_enum] -> Switch/3
  Constant52/1 -> Switch/1
  Detect Change1/1 -> Logical Operator3/1
  Logical Operator3/1 -> Logical Operator4/2
  Constant54/1 -> Equal17/2
  Logical Operator2/1 -> Logical Operator4/1
  Equal17/1 -> Logical Operator3/2
  Detect Change/1 -> Logical Operator2/1
  Logical Operator4/1 -> VPMM_DetectAntitheftUnlock_flg/1  "VPMM_DetectAntitheftUnlock_flg"
  [VBCM_AntitheftSta_enum] -> Detect Change/1, Equal18/1
  [VBCM_AntitheftSta_enum] -> Detect Change1/1, Equal17/1
  Equal18/1 -> Logical Operator2/2
  Constant53/1 -> Equal18/2
  VBCM_AntitheftSta_enum/1 -> [VBCM_AntitheftSta_enum]
  VINP_DCDCFaultSta_enum/1 -> [VINP_DCDCFaultSta_enum]
  Constant59/1 -> Equal32/2
  Constant58/1 -> Equal33/2
  [VPMM_PDKeySta_enum] -> Equal32/1, Detect Change2/1
  [VPMM_PDKeySta_enum] -> Detect Change3/1, Equal33/1
  Detect Change2/1 -> Logical Operator5/1
  Equal32/1 -> Logical Operator5/2
  Detect Change3/1 -> Logical Operator6/1
  Equal33/1 -> Logical Operator6/2
  Logical Operator5/1 -> Logical Operator7/1
  Logical Operator6/1 -> Logical Operator7/2
  Logical Operator7/1 -> VPMM_DetectPDKeyUnlock_flg/1  "VPMM_DetectPDKeyUnlock_flg"
  [VBCM_AntitheftSta_enum] -> Equal34/1, Detect Change4/1
  Detect Change4/1 -> Logical Operator8/1
  Equal34/1 -> Logical Operator8/2
  Constant60/1 -> Equal34/2
  Constant61/1 -> Equal35/2
  Equal35/1 -> Logical Operator9/2
  Detect Change5/1 -> Logical Operator9/1
  [VBCM_AntitheftSta_enum] -> Detect Change5/1, Equal35/1
  Logical Operator8/1 -> Logical Operator10/1
  Logical Operator9/1 -> Logical Operator10/2
  Logical Operator10/1 -> VPMM_DetectAntitheftLock_flg/1  "VPMM_DetectAntitheftLock_flg"
  [VPMM_PDKeySta_enum] -> Detect Change6/1, Equal36/1
  Constant62/1 -> Equal36/2
  Detect Change6/1 -> Logical Operator11/1
  Equal36/1 -> Logical Operator11/2
  Logical Operator11/1 -> VPMM_DetectPDKeyLock_flg/1  "VPMM_DetectPDKeyLock_flg"
  [task_time_s] -> Hold7/1
  Constant63/1 -> Hold7/2
  Detect Increase8/1 -> Hold7/3
  VINP_IVIPwroffreq_flg/1 -> Detect Increase8/1
  Hold7/1 -> VPMM_DetectIVIPwroffreq_flg/1  "VPMM_DetectIVIPwroffreq_flg"
  Hold8/1 -> VPMM_DetectSchedChg_flg/1  "VPMM_DetectSchedChg_flg"
  Detect Increase9/1 -> Hold8/3
  VINP_SchedChgwake_flg/1 -> Detect Increase9/1
  Constant64/1 -> Hold8/2
  [task_time_s] -> Hold8/1
  [task_time_s] -> Hold9/1
  Constant65/1 -> Hold9/2
  Detect Increase10/1 -> Hold9/3
  VINP_PWCONTINUEUSE_flg/1 -> Detect Increase10/1
  Hold9/1 -> VPMM_DetectPWCONTINUE_flg/1  "VPMM_DetectPWCONTINUE_flg"
  VINP_PDKeyAreaLockUnlock_enum/1 -> [VINP_PDKeyAreaLockUnlock_enum]
  Detect Increase11/1 -> Hold10/3
  Constant66/1 -> Hold10/2
  [task_time_s] -> Hold10/1
  VPMM_HVPwrSta_flg/1 -> Detect Increase11/1
  Hold10/1 -> VPMM_DetectHVPwrSta_flg/1  "VPMM_DetectHVPwrSta_flg"
  VINP_CrashOutputSts_enum/1 -> [VINP_CrashOutputSts_enum]
  [VINP_CrashOutputSts_enum] -> Equal/1
  Constant5/1 -> Equal/2
  Constant67/1 -> Equal37/2
  [VINP_CrashOutputSts_enum] -> Equal37/1
  [VINP_CrashOutputSts_enum] -> Equal38/1
  Constant68/1 -> Equal38/2
  NOT6/1 -> LiuzgSwitch16/1
  Constant70/1 -> LiuzgSwitch27/1
  LiuzgSwitch16/1 -> Timer/2, NOT7/1
  Constant87/1 -> NOT6/1
  Timer/1 -> Equal40/1
  [VPMM_PowerSta_enum] -> Equal41/1
  Constant76/1 -> LiuzgSwitch16/3
  Equal43/1 -> LiuzgSwitch16/2  "VPMM_TMSpdThdSta_flg"
  Constant77/1 -> Equal44/2
  Constant75/1 -> Equal40/2
  Constant69/1 -> Equal43/2
  [task_time_s] -> Timer/3
  [task_time_s] -> Timer1/3
  Equal41/1 -> LiuzgSwitch27/2
  NOT8/1 -> LiuzgSwitch17/3
  NOT7/1 -> Timer/1
  [VPMM_PowerSta_enum] -> Equal44/1
  Constant74/1 -> Timer/4
  Constant72/1 -> Equal41/2
  Equal44/1 -> LiuzgSwitch17/2
  Timer1/1 -> Equal42/1
  Equal42/1 -> NOT11/1
  Logical Operator13/1 -> NOT9/1, Timer1/1
  Equal40/1 -> NOT8/1
  NOT9/1 -> Timer1/2
  [VPMM_TMSpd_rpm] -> Equal43/1
  Constant71/1 -> Timer1/4
  NOT11/1 -> LiuzgSwitch27/3
  Constant79/1 -> Equal42/2
  Constant73/1 -> LiuzgSwitch17/1
  LiuzgSwitch27/1 -> VPMM_SafetyChkHLv_flg/1  "VPMM_SafetyChkHLv_flg"
  LiuzgSwitch17/1 -> VPMM_SafetyChkMLv_flg/1  "VPMM_SafetyChkMLv_flg"
  [VTQD_CrashDetd_flg] -> Logical Operator13/4
  Equal38/1 -> Logical Operator13/3
  Equal37/1 -> Logical Operator13/2
  Equal/1 -> Logical Operator13/1
  VINP_HVILSta_flg/1 -> Terminator4/1
  [VINP_BMSWarn6_flg] -> AND7/2
  [VINP_BMSWarn7_flg] -> AND7/3
  [VINP_BMSWarn8_flg] -> AND7/4
  VINP_BMSWarn6_flg/1 -> [VINP_BMSWarn6_flg]
  VINP_BMSWarn8_flg/1 -> [VINP_BMSWarn8_flg]
  VINP_BMSWarn7_flg/1 -> [VINP_BMSWarn7_flg]
  VINP_NewNMSpec_flg/1 -> [VINP_NewNMSpec_flg]
  VINP_VehicleType_enum/1 -> [VINP_VehicleType_enum]
  VINP_AuxBattVolmV_mV/1 -> [VINP_AuxBattVolmV_mV]
  VINP_LVBattDet12V_V/1 -> [VINP_LVBattDet12V_V]
  [VINP_DCDCFaultSta_enum] -> Terminator6/1
  From100/1 -> Gain3/1
  From99/1 -> LiuzgSwitch20/3
  [VINP_LVBattDet12V_V] -> Gain4/1
  Data Type Conversion4/1 -> VPMM_AuxBatVolt_V/1  "VPMM_AuxBatVolt_V"
  Constant35/1 -> Equal45/2
  Equal48/1 -> Switch9/1
  Gain1/1 -> VPMM_AuxBatVolt_mV_commentout/1
  Abs2/1 -> Equal48/1
  From117/1 -> Equal23/1
  Logical Operator14/1 -> LiuzgSwitch20/2, LiuzgSwitch21/2
  Timer2/1 -> Equal39/1
  Constant80/1 -> Equal46/1
  Constant36/1 -> Equal48/2
  Constant82/1 -> Switch9/3
  Logical Operator18/1 -> Logical Operator19/2  "VPMM_LVADCHiLoThdErr_flg"
  NOT1/1 -> Timer2/2
  Equal46/1 -> Logical Operator20/1
  From94/1 -> Logical Operator12/1
  Constant29/1 -> Equal19/2
  [VINP_AuxBattVolmV_mV] -> Gain5/1
  Constant57/1 -> Equal49/2
  Logical Operator19/1 -> Timer2/1, NOT1/1
  Data Type Conversion2/1 -> VPMM_AuxBatVolt_mV/1  "VPMM_AuxBatVolt_mV"
  [VINP_AuxBattVolmV_mV] -> Equal47/1
  [VPMM_PowerSta_enum] -> Unit Delay2/1
  [VINP_AuxBattVolmV_mV] -> Equal49/1
  Constant33/1 -> Equal47/2
  Equal19/1 -> Logical Operator17/2
  [VINP_CANMsgValidBMS5_flg] -> Logical Operator16/2
  Gain2/1 -> LiuzgSwitch20/1
  Equal47/1 -> Logical Operator18/1
  Equal45/1 -> Logical Operator20/2
  Switch9/1 -> Logical Operator19/1  "VPMM_LVADCDiffErr_flg"
  Add/1 -> Abs2/1
  Gain7/1 -> Add/2
  Switch7/1 -> LiuzgSwitch29/1
  [VPMM_ADCStaChkFail_flg] -> Logical Operator16/1
  Unit Delay2/1 -> Equal46/2, Equal45/1
  [VINP_NewNMSpec_flg] -> Logical Operator17/1
  Data Type Conversion1/1 -> Terminator8/1  "VPMM_AuxBatVolt_mV"
  LiuzgSwitch20/1 -> Data Type Conversion3/1
  [VINP_LVBattDet12V_V] -> Switch8/1
  Equal49/1 -> Logical Operator18/2
  Gain3/1 -> LiuzgSwitch21/3
  Constant81/1 -> Equal23/2
  Logical Operator17/1 -> LiuzgSwitch29/2, LiuzgSwitch28/2
  LiuzgSwitch29/1 -> Data Type Conversion2/1
  [VINP_AuxBattVolmV_mV] -> Add/1
  [VINP_CANMsgValidBMS5_flg] -> Switch9/2
  Gain4/1 -> Switch7/1
  Switch8/1 -> LiuzgSwitch28/1
  LiuzgSwitch19/1 -> VPMM_AuxBatVolt_V_commentout/1, Gain1/1
  Logical Operator20/1 -> SR_Latch/2
  [VINP_CANMsgValidBMS5_flg] -> Logical Operator15/2
  [VINP_LVBattDet12V_V] -> LiuzgSwitch28/3
  [task_time_s] -> Timer2/3
  Gain5/1 -> Switch8/3
  LiuzgSwitch28/1 -> Data Type Conversion4/1
  Logical Operator15/1 -> Switch7/2
  Logical Operator16/1 -> Switch8/2
  [VINP_LVBattDet12V_V] -> Gain7/1
  [VINP_LVBattDet12V_V] -> Gain6/1
  Constant78/1 -> Equal39/2
  Constant12/1 -> Equal26/2
  [VINP_AuxBattVolmV_mV] -> Switch7/3
  From97/1 -> Equal26/1
  Data Type Conversion3/1 -> Terminator7/1  "VPMM_AuxBatVolt_V"
  [VINP_VehicleType_enum] -> Equal19/1
  LiuzgSwitch21/1 -> Data Type Conversion1/1
  From102/1 -> LiuzgSwitch21/1
  [VPMM_ADCStaChkFail_flg] -> Logical Operator15/1
  Constant83/1 -> Timer2/4
  From98/1 -> Logical Operator14/1
  Equal26/1 -> Logical Operator14/2
  From101/1 -> Gain2/1
  From96/1 -> LiuzgSwitch19/3
  From95/1 -> Gain/1
  Gain/1 -> LiuzgSwitch19/1
  SR_Latch/1 -> [VPMM_ADCStaChkFail_flg]  "VPMM_ADCStaChkFail_flg"
  From93/1 -> Equal13/1
  Equal13/1 -> Logical Operator12/2
  Equal23/1 -> Terminator9/1
  Logical Operator12/1 -> LiuzgSwitch19/2
  Gain6/1 -> LiuzgSwitch29/3
  Constant10/1 -> Equal13/2
  Equal39/1 -> SR_Latch/1
  [VPMM_ADCStaChkFail_flg] -> VPMM_ADCStaChkFail_flg/1
  VINP_CANMsgValidBMS5_flg/1 -> [VINP_CANMsgValidBMS5_flg]
  Constant27/1 -> Switch1/2
  VTQD_CrashDetd_flg/1 -> [VTQD_CrashDetd_flg]
  VDDM_DrStSWCFS_flg/1 -> [VDDM_DrStSWCFS_flg]
  Switch3/1 -> Switch2/3
  Constant90/1 -> Switch2/1
  [VDDM_DrStSWCFS_flg] -> Switch2/2
  [VPMM_SeatSW_flg] -> Switch3/2
  Constant89/1 -> Switch3/3
  Constant88/1 -> Switch3/1
  Switch2/1 -> Data Type Conversion/1
  Equal50/1 -> LiuzgSwitch31/2
  AND2/1 -> Logical Operator21/1
  Equal51/1 -> LiuzgSwitch30/2
  LiuzgSwitch32/1 -> LiuzgSwitch30/3
  LiuzgSwitch30/1 -> Logical Operator22/1
  Equal52/1 -> LiuzgSwitch32/2
  [VINP_RrMCUEnaSta_flg] -> LiuzgSwitch32/1
  [VPMM_DrivetrainSelect_enum] -> Equal51/1
  [VPMM_DrivetrainSelect_enum] -> Equal52/1
  Logical Operator22/1 -> LiuzgSwitch31/3
  [VINP_RrMCUEnaSta_flg] -> AND2/2
  Constant85/1 -> Equal51/2
  [VPMM_DrivetrainSelect_enum] -> Equal50/1
  Constant55/1 -> LiuzgSwitch32/3
  Logical Operator21/1 -> LiuzgSwitch31/1
  Constant86/1 -> Equal52/2
  Constant84/1 -> Equal50/2
  [VINP_FrMCUEnaSta_flg] -> AND2/1
  [VINP_FrMCUEnaSta_flg] -> LiuzgSwitch30/1
  LiuzgSwitch31/1 -> VPMM_MCUDisable_flg/1  "VPMM_MCUDisable_flg"
  LiuzgSwitch14/1 -> Switch4/3
  Switch4/1 -> [VPMM_PDKeySta_enum], VPMM_PDKeySta_enum/1  "VPMM_PDKeySta_enum"
  Constant42/1 -> Switch4/1
  Constant44/1 -> Switch4/2
  [task_time_s] -> DelayEnable/3
  Constant91/1 -> DelayEnable/2
  DelayEnable/1 -> [VPMM_SeatOccupyCheck_flg]
  [task_time_s] -> DelayEnable1/3
  Constant92/1 -> DelayEnable1/2
  Logical Operator/1 -> DelayEnable1/1
  Delay/1 -> SR_Latch1/2
  [VPMM_SeatEmptyCheck_flg] -> Delay/1
  SR_Latch1/1 -> Switch5/2
  [VPMM_SeatOccupyCheck_flg] -> SR_Latch1/1
  Switch5/1 -> [VPMM_SeatEmptyCheck_flg]
  DelayEnable1/1 -> Switch5/1
  Constant93/1 -> Switch5/3
  [VPMM_SeatOccupyCheck_flg] -> SR_Latch2/1
  [VPMM_SeatEmptyCheck_flg] -> SR_Latch2/2
  SR_Latch2/1 -> Detect Increase6/1

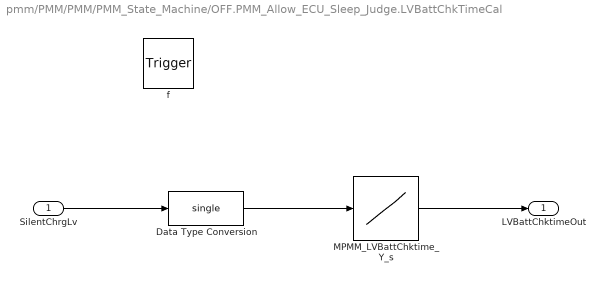
== system pmm/PMM/PMM/PMM_State_Machine/OFF.PMM_Allow_ECU_Sleep_Judge.LVBattChkTimeCal ==
  SilentChrgLv : Inport
  f : TriggerPort  TriggerType=function-call  VariantControl=(inherit)
      settings: CopyFcn=Stateflow.SLINSF.SimulinkMan.removeBlockPreDeleteFcn  PreDeleteFcn=Stateflow.SLINSF.SimulinkMan.unsafePredeleteFcn
  Data Type Conversion : DataTypeConversion  OutDataTypeStr=single
  MPMM_LVBattChktime_Y_s : Lookup_n-D  NumberOfTableDimensions=1  BreakpointsForDimension1=APMM_LVBattChktime_X_enum  Table=MPMM_LVBattChktime_Y_s  ExtrapMethod=Clip  InternalRulePriority=Speed  RndMeth=Simplest  InputSameDT=on
  LVBattChktimeOut : Outport
  wires:
  MPMM_LVBattChktime_Y_s/1 -> LVBattChktimeOut/1
  SilentChrgLv/1 -> Data Type Conversion/1
  Data Type Conversion/1 -> MPMM_LVBattChktime_Y_s/1

== system pmm/PMM/PMM/PMM_State_Machine/OFF.Silent_Charge_Judge.SilentChrgLvCal ==
  LVBatt_mV : Inport
  f : TriggerPort  TriggerType=function-call  VariantControl=(inherit)
      settings: CopyFcn=Stateflow.SLINSF.SimulinkMan.removeBlockPreDeleteFcn  PreDeleteFcn=Stateflow.SLINSF.SimulinkMan.unsafePredeleteFcn
  MPMM_LVChrgLv_Y_Lv : Lookup_n-D  NumberOfTableDimensions=1  BreakpointsForDimension1=APMM_LVChrgLv_X_mV  Table=MPMM_LVChrgLv_Y_Lv  ExtrapMethod=Clip  InternalRulePriority=Speed  RndMeth=Simplest  InputSameDT=on
  SilentChrgLv : Outport
  wires:
  MPMM_LVChrgLv_Y_Lv/1 -> SilentChrgLv/1  "VPMM_LVChrgLvOut_enum"
  LVBatt_mV/1 -> MPMM_LVChrgLv_Y_Lv/1

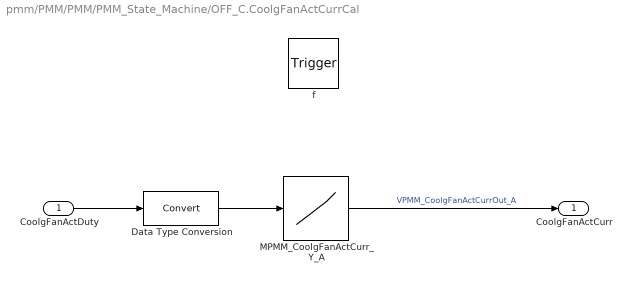
== system pmm/PMM/PMM/PMM_State_Machine/OFF_C.CoolgFanActCurrCal ==
  CoolgFanActDuty : Inport
  f : TriggerPort  TriggerType=function-call  VariantControl=(inherit)
      settings: CopyFcn=Stateflow.SLINSF.SimulinkMan.removeBlockPreDeleteFcn  PreDeleteFcn=Stateflow.SLINSF.SimulinkMan.unsafePredeleteFcn
  Data Type Conversion : DataTypeConversion
  MPMM_CoolgFanActCurr_Y_A : Lookup_n-D  NumberOfTableDimensions=1  BreakpointsForDimension1=APMM_CoolgFanActCurr_X_pct  Table=MPMM_CoolgFanActCurr_Y_A  ExtrapMethod=Clip  InternalRulePriority=Speed  RndMeth=Simplest  InputSameDT=on
  CoolgFanActCurr : Outport
  wires:
  MPMM_CoolgFanActCurr_Y_A/1 -> CoolgFanActCurr/1  "VPMM_CoolgFanActCurrOut_A"
  CoolgFanActDuty/1 -> Data Type Conversion/1
  Data Type Conversion/1 -> MPMM_CoolgFanActCurr_Y_A/1

== system pmm/PMM/PMM/PMM_State_Machine/OFF_C.EWP1CurrCal ==
  FDEWP1Cmd : Inport
  f : TriggerPort  TriggerType=function-call  VariantControl=(inherit)
      settings: CopyFcn=Stateflow.SLINSF.SimulinkMan.removeBlockPreDeleteFcn  PreDeleteFcn=Stateflow.SLINSF.SimulinkMan.unsafePredeleteFcn
  Data Type Conversion : DataTypeConversion
  MPMM_EWP1Curr_Y_A : Lookup_n-D  NumberOfTableDimensions=1  BreakpointsForDimension1=APMM_EWP1Curr_X_c  Table=MPMM_EWP1Curr_Y_A  ExtrapMethod=Clip  InternalRulePriority=Speed  RndMeth=Simplest  InputSameDT=on
  EWP1Curr : Outport
  wires:
  MPMM_EWP1Curr_Y_A/1 -> EWP1Curr/1  "VPMM_EWP1CurrOut_A"
  FDEWP1Cmd/1 -> Data Type Conversion/1
  Data Type Conversion/1 -> MPMM_EWP1Curr_Y_A/1

== system pmm/PMM/PMM/PMM_State_Machine/OFF_C.EWP3CurrCal ==
  FDEWP3Cmd : Inport
  f : TriggerPort  TriggerType=function-call  VariantControl=(inherit)
      settings: CopyFcn=Stateflow.SLINSF.SimulinkMan.removeBlockPreDeleteFcn  PreDeleteFcn=Stateflow.SLINSF.SimulinkMan.unsafePredeleteFcn
  Data Type Conversion : DataTypeConversion
  MPMM_EWP3Curr_Y_A : Lookup_n-D  NumberOfTableDimensions=1  BreakpointsForDimension1=APMM_EWP3Curr_X_c  Table=MPMM_EWP3Curr_Y_A  ExtrapMethod=Clip  InternalRulePriority=Speed  RndMeth=Simplest  InputSameDT=on
  EWP3Curr : Outport
  wires:
  MPMM_EWP3Curr_Y_A/1 -> EWP3Curr/1  "VPMM_EWP3CurrOut_A"
  FDEWP3Cmd/1 -> Data Type Conversion/1
  Data Type Conversion/1 -> MPMM_EWP3Curr_Y_A/1

== system pmm/PMM/PMM/PMM_State_Machine/OFF_C.LVBattChrgTimeCal ==
  SilentChrgLv : Inport
  f : TriggerPort  TriggerType=function-call  VariantControl=(inherit)
      settings: CopyFcn=Stateflow.SLINSF.SimulinkMan.removeBlockPreDeleteFcn  PreDeleteFcn=Stateflow.SLINSF.SimulinkMan.unsafePredeleteFcn
  MPMM_LVBattChrgtime_Y_s : Lookup_n-D  NumberOfTableDimensions=1  BreakpointsForDimension1=APMM_LVBattChrgtime_X_enum  Table=MPMM_LVBattChrgtime_Y_s  ExtrapMethod=Clip  InternalRulePriority=Speed  RndMeth=Simplest  InputSameDT=on
  LVBattChrgTime : Outport
  wires:
  MPMM_LVBattChrgtime_Y_s/1 -> LVBattChrgTime/1  "VPMM_LVBattChrgtimeOut_s"
  SilentChrgLv/1 -> MPMM_LVBattChrgtime_Y_s/1

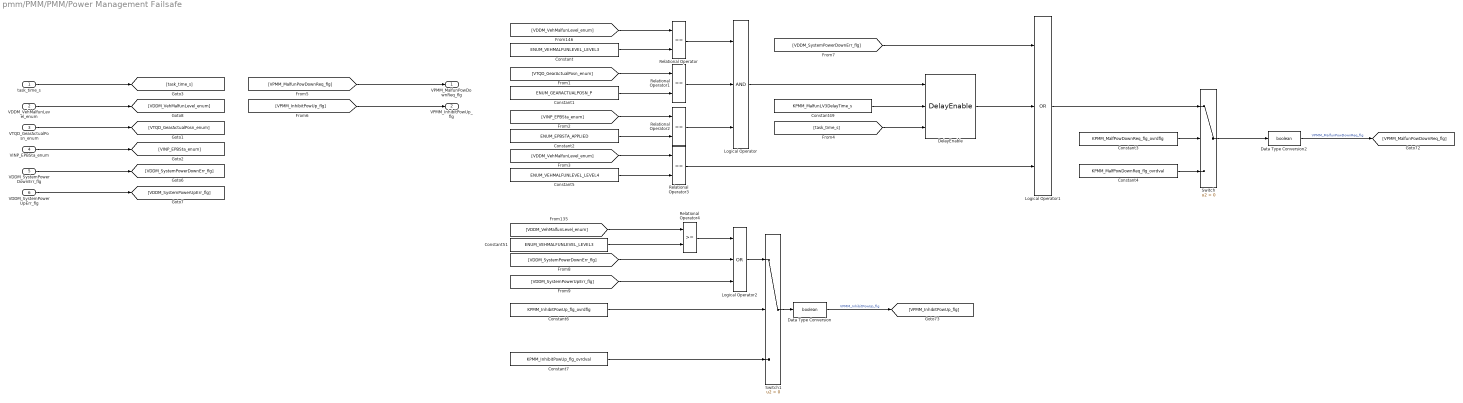
== system pmm/PMM/PMM/Power Management Failsafe ==
  task_time_s : Inport
  VDDM_VehMalfunLevel_enum : Inport  Port=2
  VTQD_GearActualPosn_enum : Inport  Port=3
  VINP_EPBSta_enum : Inport  Port=4
  VDDM_SystemPowerDownErr_flg : Inport  Port=5
  VDDM_SystemPowerUpErr_flg : Inport  Port=6
  Constant : Constant  Value=ENUM_VEHMALFUNLEVEL_LEVEL3
  Constant1 : Constant  Value=ENUM_GEARACTUALPOSN_P
  Constant2 : Constant  Value=ENUM_EPBSTA_APPLIED
  Constant3 : Constant  Value=KPMM_MalfPowDownReq_flg_ovrdflg
  Constant4 : Constant  Value=KPMM_MalfPowDownReq_flg_ovrdval
  Constant49 : Constant  Value=KPMM_MalfunLV3DelayTime_s
  Constant5 : Constant  Value=ENUM_VEHMALFUNLEVEL_LEVEL4
  Constant51 : Constant  Value=ENUM_VEHMALFUNLEVEL_LEVEL3
  Constant6 : Constant  Value=KPMM_InhibitPowUp_flg_ovrdflg
  Constant7 : Constant  Value=KPMM_InhibitPowUp_flg_ovrdval
  Data Type Conversion : DataTypeConversion  OutDataTypeStr=boolean
  Data Type Conversion2 : DataTypeConversion  OutDataTypeStr=boolean
  DelayEnable : hcu_lib/Basic_Blocks/DelayEnable
  Logical Operator : Logic  Inputs=3  AllPortsSameDT=off  OutDataTypeStr=boolean
  Logical Operator1 : Logic  Operator=OR  Inputs=3  AllPortsSameDT=off  OutDataTypeStr=boolean
  Logical Operator2 : Logic  Operator=OR  Inputs=3  AllPortsSameDT=off  OutDataTypeStr=boolean
  Relational Operator{,1..3} (4 alike) : RelationalOperator  Operator===  OutDataTypeStr=boolean  RndMeth=Simplest
  Relational Operator4 : RelationalOperator  OutDataTypeStr=boolean  RndMeth=Simplest
  Switch : Switch  Criteria=u2 > Threshold
  Switch1 : Switch  Criteria=u2 > Threshold
  VPMM_MalfunPowDownReq_flg : Outport
  VPMM_InhibitPowUp_flg : Outport  Port=2
  wires:
  VDDM_VehMalfunLevel_enum/1 -> [VDDM_VehMalfunLevel_enum]
  VTQD_GearActualPosn_enum/1 -> [VTQD_GearActualPosn_enum]
  VINP_EPBSta_enum/1 -> [VINP_EPBSta_enum]
  task_time_s/1 -> [task_time_s]
  Relational Operator/1 -> Logical Operator/1
  [VDDM_VehMalfunLevel_enum] -> Relational Operator/1
  Constant/1 -> Relational Operator/2
  Relational Operator1/1 -> Logical Operator/2
  [VTQD_GearActualPosn_enum] -> Relational Operator1/1
  Constant1/1 -> Relational Operator1/2
  Relational Operator2/1 -> Logical Operator/3
  [VINP_EPBSta_enum] -> Relational Operator2/1
  Constant2/1 -> Relational Operator2/2
  Constant3/1 -> Switch/2
  Switch/1 -> Data Type Conversion2/1
  [VDDM_VehMalfunLevel_enum] -> Relational Operator3/1
  Constant5/1 -> Relational Operator3/2
  Logical Operator/1 -> DelayEnable/1
  Constant49/1 -> DelayEnable/2
  [task_time_s] -> DelayEnable/3
  Relational Operator3/1 -> Logical Operator1/3
  Switch1/1 -> Data Type Conversion/1
  Constant6/1 -> Switch1/2
  [VDDM_VehMalfunLevel_enum] -> Relational Operator4/1
  Constant51/1 -> Relational Operator4/2
  Constant7/1 -> Switch1/3
  Constant4/1 -> Switch/3
  Logical Operator1/1 -> Switch/1
  [VPMM_MalfunPowDownReq_flg] -> VPMM_MalfunPowDownReq_flg/1
  [VPMM_InhibitPowUp_flg] -> VPMM_InhibitPowUp_flg/1
  Data Type Conversion/1 -> [VPMM_InhibitPowUp_flg]  "VPMM_InhibitPowUp_flg"
  Data Type Conversion2/1 -> [VPMM_MalfunPowDownReq_flg]  "VPMM_MalfunPowDownReq_flg"
  VDDM_SystemPowerUpErr_flg/1 -> [VDDM_SystemPowerUpErr_flg]
  VDDM_SystemPowerDownErr_flg/1 -> [VDDM_SystemPowerDownErr_flg]
  DelayEnable/1 -> Logical Operator1/2
  [VDDM_SystemPowerDownErr_flg] -> Logical Operator1/1
  Logical Operator2/1 -> Switch1/1
  Relational Operator4/1 -> Logical Operator2/1
  [VDDM_SystemPowerDownErr_flg] -> Logical Operator2/2
  [VDDM_SystemPowerUpErr_flg] -> Logical Operator2/3

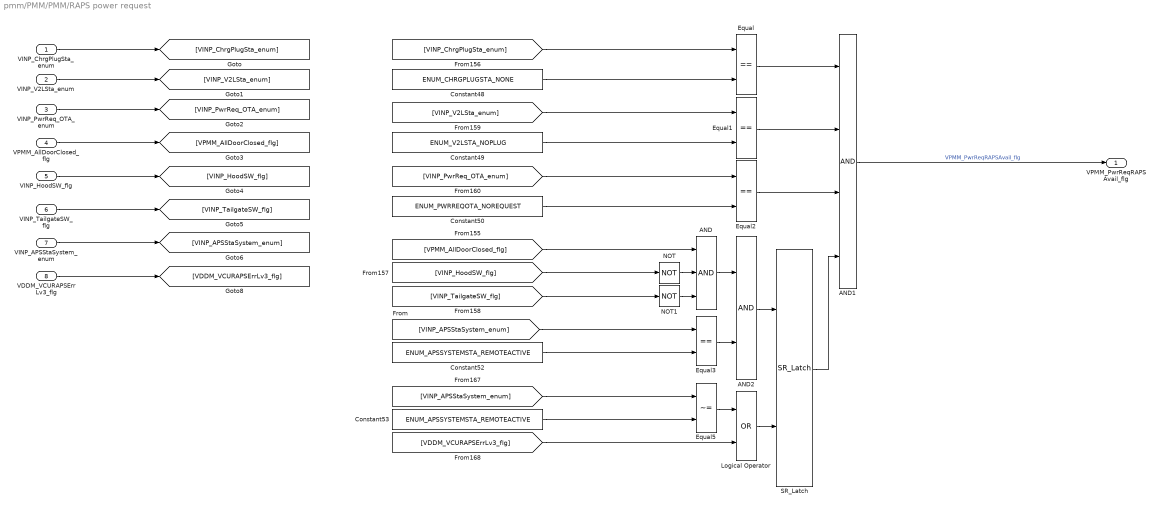
== system pmm/PMM/PMM/RAPS power request ==
  VINP_ChrgPlugSta_enum : Inport
  VINP_V2LSta_enum : Inport  Port=2
  VINP_PwrReq_OTA_enum : Inport  Port=3
  VPMM_AllDoorClosed_flg : Inport  Port=4
  VINP_HoodSW_flg : Inport  Port=5
  VINP_TailgateSW_flg : Inport  Port=6
  VINP_APSStaSystem_enum : Inport  Port=7
  VDDM_VCURAPSErrLv3_flg : Inport  Port=8
  AND : Logic  Inputs=3  AllPortsSameDT=off  OutDataTypeStr=boolean
  AND1 : Logic  Inputs=4  AllPortsSameDT=off  OutDataTypeStr=boolean
  AND2 : Logic  AllPortsSameDT=off  OutDataTypeStr=boolean
  Constant48 : Constant  Value=ENUM_CHRGPLUGSTA_NONE
  Constant49 : Constant  Value=ENUM_V2LSTA_NOPLUG
  Constant50 : Constant  Value=ENUM_PWRREQOTA_NOREQUEST
  Constant52 : Constant  Value=ENUM_APSSYSTEMSTA_REMOTEACTIVE
  Constant53 : Constant  Value=ENUM_APSSYSTEMSTA_REMOTEACTIVE
  Equal{,1..3} (4 alike) : RelationalOperator  Operator===  OutDataTypeStr=boolean  RndMeth=Simplest
  Equal5 : RelationalOperator  Operator=~=  OutDataTypeStr=boolean  RndMeth=Simplest
  Logical Operator : Logic  Operator=OR  AllPortsSameDT=off  OutDataTypeStr=boolean
  NOT : Logic  Operator=NOT  AllPortsSameDT=off  OutDataTypeStr=boolean
  NOT1 : Logic  Operator=NOT  AllPortsSameDT=off  OutDataTypeStr=boolean
  SR_Latch : hcu_lib/Basic_Blocks/SR_Latch
  VPMM_PwrReqRAPSAvail_flg : Outport
  wires:
  Equal3/1 -> AND2/2
  [VPMM_AllDoorClosed_flg] -> AND/1
  Constant52/1 -> Equal3/2
  Constant50/1 -> Equal2/2
  NOT1/1 -> AND/3
  Constant53/1 -> Equal5/2
  AND1/1 -> VPMM_PwrReqRAPSAvail_flg/1  "VPMM_PwrReqRAPSAvail_flg"
  Constant48/1 -> Equal/2
  Equal5/1 -> Logical Operator/1
  [VINP_PwrReq_OTA_enum] -> Equal2/1
  [VINP_ChrgPlugSta_enum] -> Equal/1
  [VINP_TailgateSW_flg] -> NOT1/1
  Constant49/1 -> Equal1/2
  AND/1 -> AND2/1
  [VINP_V2LSta_enum] -> Equal1/1
  [VINP_APSStaSystem_enum] -> Equal5/1
  Equal/1 -> AND1/1
  [VINP_HoodSW_flg] -> NOT/1
  NOT/1 -> AND/2
  Equal2/1 -> AND1/3
  [VINP_APSStaSystem_enum] -> Equal3/1
  AND2/1 -> SR_Latch/1
  Equal1/1 -> AND1/2
  SR_Latch/1 -> AND1/4
  VINP_ChrgPlugSta_enum/1 -> [VINP_ChrgPlugSta_enum]
  VINP_V2LSta_enum/1 -> [VINP_V2LSta_enum]
  VINP_PwrReq_OTA_enum/1 -> [VINP_PwrReq_OTA_enum]
  VPMM_AllDoorClosed_flg/1 -> [VPMM_AllDoorClosed_flg]
  VINP_HoodSW_flg/1 -> [VINP_HoodSW_flg]
  VINP_TailgateSW_flg/1 -> [VINP_TailgateSW_flg]
  VINP_APSStaSystem_enum/1 -> [VINP_APSStaSystem_enum]
  [VDDM_VCURAPSErrLv3_flg] -> Logical Operator/2
  Logical Operator/1 -> SR_Latch/2
  VDDM_VCURAPSErrLv3_flg/1 -> [VDDM_VCURAPSErrLv3_flg]
